simulink model "Labo2parte1"  (R2025b)
settings: Solver=FixedStepAuto  StartTime=0.0  StopTime=40  RelTol=1e-3  EnableMultiTasking=on
libraries: arduinolib x6, arduinosensorlib x1
settings Model: ExtModeTrigDuration=2  Creator=ALIENWARE-GAMER  LastModifiedBy=Froilán Pardo
settings SolverCC: AutoInsertRateTranBlk=on
settings OptimizationCC: BlockReduction=off  BooleanDataType=off  EnhancedBackFolding=on  PassReuseOutputArgsAs=Individual arguments  ZeroExternalMemoryAtStartup=off  ZeroInternalMemoryAtStartup=off  MaxStackSize=64  OptimizeBlockOrder=speed  DifferentSizesBufferReuse=on  OptimizationCustomize=off  EfficientTunableParamExpr=on
settings DebuggingCC: SaveWithParameterizedLinksMsg=none  UnderspecifiedInitializationDetection=Classic  MergeDetectMultiDrivingBlocksExec=none  SignalResolutionControl=TryResolveAllWithWarning  ParameterTunabilityLossMsg=error
settings HardwareCC: ProdBitPerInt=16.0  ProdBitPerPointer=16.0  ProdBitPerSizeT=16.0  ProdBitPerPtrDiffT=16.0  ProdLargestAtomicFloat=None  ProdWordSize=8.0  ProdHWDeviceType=Atmel->AVR  TargetBitPerInt=16.0  TargetBitPerPointer=16.0  TargetBitPerSizeT=16.0  TargetBitPerPtrDiffT=16.0  TargetIntDivRoundTo=Zero  TargetEndianess=LittleEndian  TargetWordSize=8.0  TargetHWDeviceType=Atmel->AVR
settings ModelReferenceCC: PropagateSignalLabelsOutOfModel=off
settings SFSimCC: MATLABDynamicMemAlloc=off
settings RTWCC: SystemTargetFile=ert.tlc  HardwareBoard=Arduino Uno  TemplateMakefile=ert_default_tmf  Toolchain=Arduino AVR  BuildConfiguration=Faster Runs  Description=Embedded Coder
settings CodeAppCC: ForceParamTrailComments=on  IgnoreCustomStorageClasses=off  OperatorAnnotations=on  SimulinkDataObjDesc=on  SFDataObjDesc=on  InsertBlockDesc=on
settings ERTTargetCC: ExtModeTransport=3.0  ExtModeStaticAlloc=on  ExtModeAutomaticAllocSize=off  ExtModeStaticAllocSize=250.0  ExtModeMexFile=ext_xcp  ExtModeIntrfLevel=Level2 - Open  InlinedParameterPlacement=Hierarchical  SupportContinuousTime=on  SupportVariableSizeSignals=on

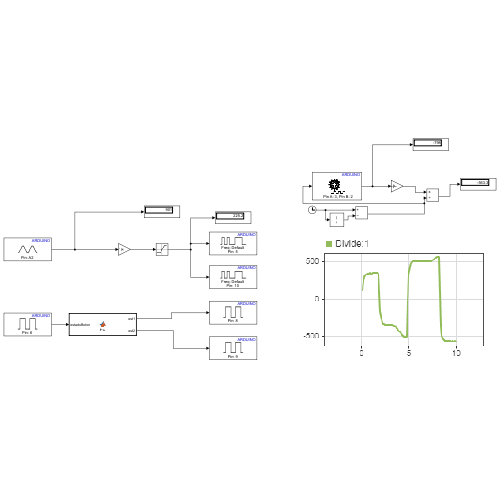
[thumbnail: Simulink's stored preview of the top-level diagram]
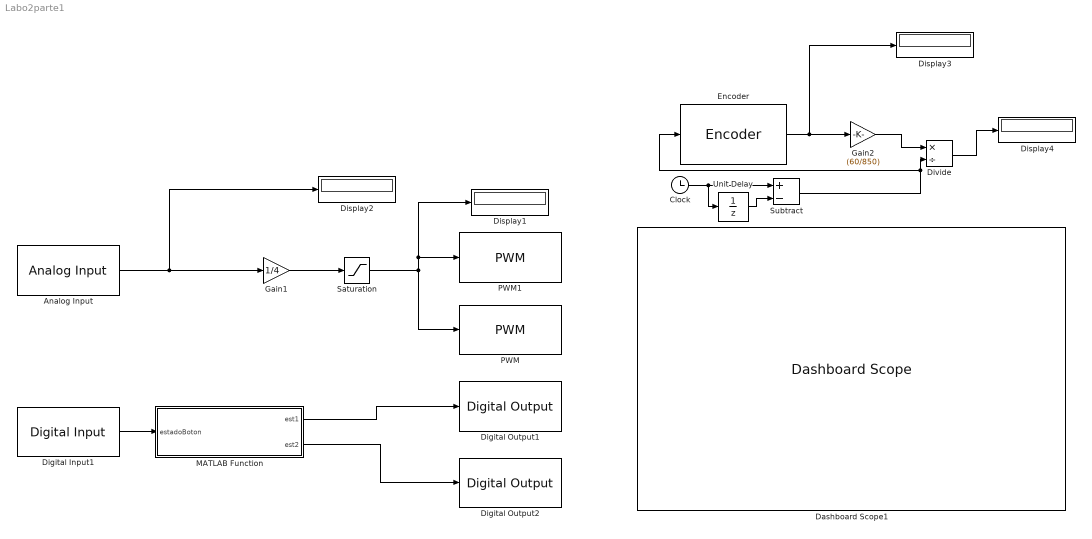
== system Labo2parte1 ==
  Analog Input : arduinolib/Analog Input  pinNumber=2  ReadResultsOnly=off  ConversionTriggerSource=Software  ExternalTriggerType=uint32( 0 )  OutputDataType=uint16  EnableConversionCompleteNotify=off  EnableOuputStatus=off  SampleTime=-1  blockPlatform=arduino
  Clock : Clock
  Dashboard Scope1 : DashboardScope  Ymin=0  Ymax=1000  FontColor=[0.0, 0.0, 0.0]
  Digital Input1 : arduinolib/Digital Input  pinNumber=6  mode=Default  Direction=input  SampleTime=0.1  blockPlatform=arduino
  Digital Output1 : arduinolib/Digital Output  pinNumber=8  Direction=output  blockPlatform=arduino
  Digital Output2 : arduinolib/Digital Output  pinNumber=9  Direction=output  blockPlatform=arduino
  Display{1..4} (4 alike) : Display
  Divide : Product  Inputs=*/
  Encoder : arduinosensorlib/Encoder  InputA=3  InputB=2  Mode=Reset by external signal  SampleTime=-1
  Gain1 : Gain  Gain=1/4
  Gain2 : Gain  Gain=(60/850)
  MATLAB Function : MATLAB Function  TreatAsAtomicUnit=on
  PWM : arduinolib/PWM  pinNumber=10  frequencyType=Default  desiredFrequency=490.2  achievableFrequency=490.2
  PWM1 : arduinolib/PWM  pinNumber=5  frequencyType=Default  desiredFrequency=490.2  achievableFrequency=490.2
  Saturation : Saturate  UpperLimit=255  LowerLimit=0
  Subtract : Sum  Inputs=+-
  Unit Delay : UnitDelay  SampleTime=-1  HasFrameUpgradeWarning=on
  wires:
  Gain1/1 -> Saturation/1
  Analog Input/1 -> Gain1/1, Display2/1
  Saturation/1 -> PWM1/1, Display1/1, PWM/1
  Digital Input1/1 -> MATLAB Function/1(estadoBoton)
  MATLAB Function/1(est1) -> Digital Output1/1
  MATLAB Function/2(est2) -> Digital Output2/1
  Encoder/1 -> Gain2/1, Display3/1
  Subtract/1 -> Divide/2, Encoder/1
  Unit Delay/1 -> Subtract/2
  Clock/1 -> Subtract/1, Unit Delay/1
  Gain2/1 -> Divide/1
  Divide/1 -> Display4/1

== matlab function Labo2parte1/MATLAB Function ==
  data: estadoBoton input; est1 output; est2 output
function [est1, est2] = fcn(estadoBoton)

persistent estadoAnterior
persistent est1_mem
persistent est2_mem

if isempty(estadoAnterior)
    estadoAnterior = 0;
end

if isempty(est1_mem)
    est1_mem = 1;
end

if isempty(est2_mem)
    est2_mem = 0;
end

% Detectar una nueva pulsación: 0 -> 1
if estadoBoton == 1 && estadoAnterior == 0

    % Intercambiar est1 y est2
    aux = est2_mem;
    est2_mem = est1_mem;
    est1_mem = aux;

end

% Guardar estado anterior del botón
estadoAnterior = double(estadoBoton);

% Salidas
est1 = est1_mem;
est2 = est2_mem;
